simulink model "Schloss_Alarm_Box"  (R2019b)
settings: Solver=FixedStepAuto  StartTime=0.0  StopTime=10.0  RelTol=1e-3
PreLoadFcn:
  | waijung.modelPreload; % Required for working with Waijung Blockset. Do not remove.
undefined symbols (not defined in the file): HSEOSC, Link, LQFP176, ST, STM32F417IG
libraries: canmsglib x8, stm32f4_canbus_lib x4, simulink x2, stm32f4_io_lib x2, stm32f4_device_config_lib x1
CloseFcn:
  | waijung.modelClose; % Required for working with Waijung Blockset. Do not remove.
settings Model: Creator=id605605  LastModifiedBy=MichaelRogalski
settings OptimizationCC: DefaultParameterBehavior=Inlined  EnhancedBackFolding=on  PassReuseOutputArgsAs=Individual arguments  ZeroExternalMemoryAtStartup=off  ZeroInternalMemoryAtStartup=off  OptimizeBlockOrder=speed  DifferentSizesBufferReuse=on  OptimizationCustomize=off  EfficientTunableParamExpr=on
settings DebuggingCC: ParameterTunabilityLossMsg=error  ArithmeticOperatorsInVariantConditions=warning
settings HardwareCC: ProdBitPerPointer=32  ProdBitPerSizeT=32  ProdBitPerPtrDiffT=32  ProdLargestAtomicFloat=None  ProdIntDivRoundTo=Undefined  ProdWordSize=32  ProdHWDeviceType=ARM Compatible->Cortex - M4  TargetEndianess=LittleEndian  TargetHWDeviceType=ARM Compatible->Cortex - M4
settings SFSimCC: MATLABDynamicMemAlloc=off  CustomCodeUndefinedFunction=UseInterfaceOnly
settings RTWCC: Description=STM32F4 Target  SystemTargetFile=stm32f4.tlc  GenerateMakefile=off  TemplateMakefile=ert_default_tmf  GenerateReport=on  IncludeHyperlinkInReport=on  LaunchReport=on  GenerateTraceInfo=on  GenerateTraceReport=on  GenerateTraceReportSl=on  GenerateTraceReportSf=on  GenerateTraceReportEml=on
settings CodeAppCC: ForceParamTrailComments=on  IgnoreCustomStorageClasses=off  OperatorAnnotations=on  SimulinkDataObjDesc=on  SFDataObjDesc=on  InsertBlockDesc=on
settings STFCustomTargetCC: TargetLangStandard=C99 (ISO)  MultiwordLength=256  ModelReferenceCompliant=off  CombineOutputUpdateFcns=on  ERTCustomFileBanners=on  SupportContinuousTime=off  SupportNonInlinedSFcns=off  RemoveResetFunc=on  MATLABClassNameForMDSCustomization=Simulink.SoftwareTarget.ERTCustomization  SystemTargetFile=stm32f4.tlc
settings ERTTargetCC: TargetLangStandard=C99 (ISO)  ModelReferenceCompliant=off  ParMdlRefBuildCompliant=off  CompOptLevelCompliant=off  ConcurrentExecutionCompliant=off  ModelStepFunctionPrototypeControlCompliant=off  CPPClassGenCompliant=off  UseToolchainInfoCompliant=off  InlinedParameterPlacement=NonHierarchical  ERTSrcFileBannerTemplate=stm32f4_code_template.cgt  ERTHdrFileBannerTemplate=stm32f4_code_template.cgt  ERTDataSrcFileTemplate=stm32f4_code_template.cgt  ERTDataHdrFileTemplate=stm32f4_code_template.cgt  ERTCustomFileTemplate=stm32f4_file_process.tlc

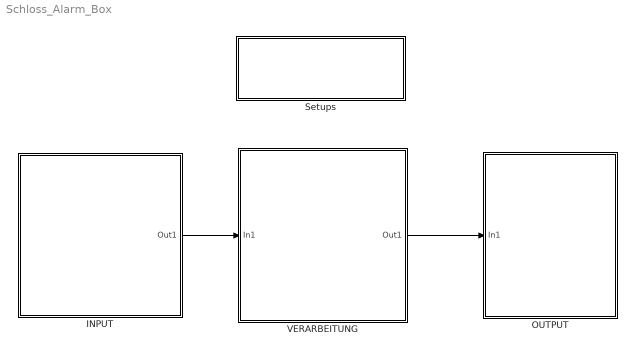
== system Schloss_Alarm_Box ==
  INPUT : Subsystem
  OUTPUT : Subsystem
  Setups : Subsystem
  VERARBEITUNG : Subsystem
  wires:
  INPUT/1(Out1) -> VERARBEITUNG/1(In1)
  VERARBEITUNG/1(Out1) -> OUTPUT/1(In1)

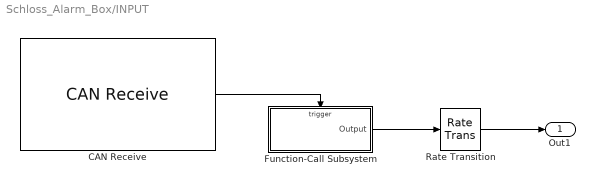
== system Schloss_Alarm_Box/INPUT ==
  CAN Receive : stm32f4_canbus_lib/CAN Receive  conf=Rx  canmodule=1  idtype=Standard  filtertype=Mask  id=0  idmask=0  enableisr=on  usedlc=off  datatype=single  data0type=uint32  data1type=uint32  data2type=Not used  data3type=Not used  data4type=Not used  data5type=Not used  data6type=Not used  data7type=Not used  buffersize=8  sampletime=-1  sampletimestr=-1  blockid=INPUTCANReceive  inputarray=[]  inputlabelarray={}  outputarray=[7]  outputlabelarray={'Call ISR' }  compat=0  confstr=[]
      settings: SourceProductName=Waijung Blockset
  Function-Call Subsystem : Subsystem  TreatAsAtomicUnit=on
  Rate Transition : RateTransition
  Out1 : Outport  VectorParamsAs1DForOutWhenUnconnected=off
  wires:
  CAN Receive/1 -> Function-Call Subsystem/Trigger
  Function-Call Subsystem/1(Output) -> Rate Transition/1
  Rate Transition/1 -> Out1/1

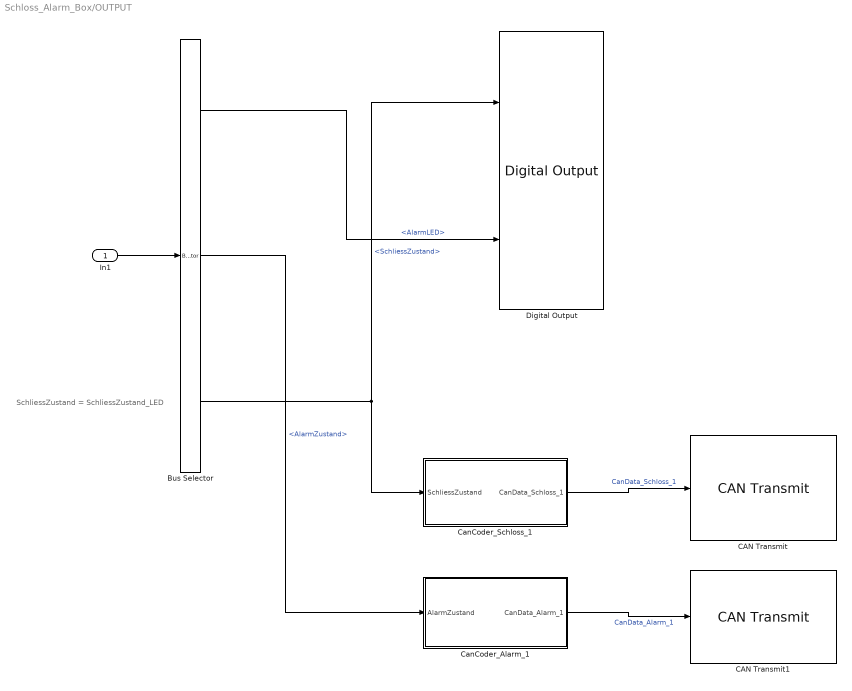
== system Schloss_Alarm_Box/OUTPUT ==
  note: SchliessZustand = SchliessZustand_LED
  In1 : Inport
  Bus Selector : BusSelector  OutputSignals=AlarmLED,AlarmZustand,SchliessZustand
  CAN Transmit : stm32f4_canbus_lib/CAN Transmit  conf=Tx  canmodule=1  transfer=Blocking  timeout=0.005  idtype=Standard  specificid=on  id=25  specificdlc=on  dlc=1  enablestatus=off  datatype=single  data0type=uint8  data1type=Not used  data2type=Not used  data3type=Not used  data4type=Not used  data5type=Not used  data6type=Not used  data7type=Not used  inputarray=[ 3]  inputlabelarray={ 'D0 (uint8)' }  outputarray=[]  outputlabelarray={}  sampletime=-1  sampletimestr=-1  blockid=OUTPUTCANTransmit  compat=0  confstr=[]
  CAN Transmit1 : stm32f4_canbus_lib/CAN Transmit  conf=Tx  canmodule=1  transfer=Blocking  timeout=0.005  idtype=Standard  specificid=on  id=24  specificdlc=on  dlc=1  enablestatus=off  datatype=single  data0type=uint8  data1type=Not used  data2type=Not used  data3type=Not used  data4type=Not used  data5type=Not used  data6type=Not used  data7type=Not used  inputarray=[ 3]  inputlabelarray={ 'D0 (uint8)' }  outputarray=[]  outputlabelarray={}  sampletime=-1  sampletimestr=-1  blockid=OUTPUTCANTransmit1  compat=0  confstr=[]
  CanCoder_Alarm_1 : Subsystem
  CanCoder_Schloss_1 : Subsystem
  Digital Output : stm32f4_io_lib/Digital Output  use_bitband=on  port=C  speed=100  porttype=Push Pull  porttypestr=PP  use_pin0=off  use_pin1=off  use_pin2=on  use_pin3=on  use_pin4=off  use_pin5=off  use_pin6=off  use_pin7=off  use_pin8=off  use_pin9=off  use_pin10=off  use_pin11=off  use_pin12=off  use_pin13=off  use_pin14=off  use_pin15=off  pinstr=GPIO_Pin_2 | GPIO_Pin_3  usedpinarray="[0  0  1  1  0  0  0  0  0  0  0  0  0  0  0  0]"  bitbandingstr=|  sampletime=-1  sampletimestr=-1  blockid=OUTPUTDigitalOutput  enablecustomportlabel=off  globalinit=off  cinputportlabel=In1, In2  coutputportlabel=0
      | #define OUTPUTDigitalOutput_C2 Peripheral_BB(GPIOC->ODR, 2)  /* Output pin */
      | #define OUTPUTDigitalOutput_C3 Peripheral_BB(GPIOC->ODR, 3)  /* Output pin */
      settings: SourceProductName=Waijung Blockset
  wires:
  In1/1 -> Bus Selector/1
  Bus Selector/1 -> Digital Output/2  "<AlarmLED>"
  Bus Selector/2 -> CanCoder_Alarm_1/1(AlarmZustand)  "<AlarmZustand>"
  Bus Selector/3 -> Digital Output/1, CanCoder_Schloss_1/1(SchliessZustand)  "<SchliessZustand>"
  CanCoder_Schloss_1/1(CanData_Schloss_1) -> CAN Transmit/1  "CanData_Schloss_1"
  CanCoder_Alarm_1/1(CanData_Alarm_1) -> CAN Transmit1/1  "CanData_Alarm_1"

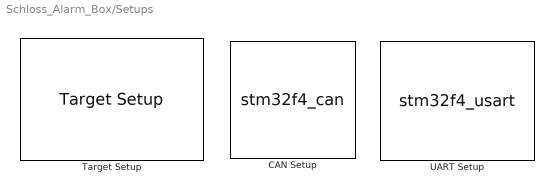
== system Schloss_Alarm_Box/Setups ==
  CAN Setup : S-Function  FunctionName=stm32f4_can  Parameters=conf,canmodule,0,inputarray,outputarray,'','',confstr,sampletime,sampletimestr,blockid  SFunctionDeploymentMode=off  EnableBusSupport=off  mask(stm32f4_can){conf=Setup, canmodule=1, advance=off, bitrate_select=500000, sjw=1tq, bs1=14tq, bs2=6tq, timingconf=Prescaler, brp=4, bitrate=500000, tq=9.5238e-08, autoretransmission=Disable, remaptxpin=A12, remaprxpin=A11, sampletime=-1, sampletimestr=-1, blockid=SetupsCANSetup, inputarray=[], inputlabelarray={}, outputarray=[], outputlabelarray={}, compat=0, confstr=[], presc=4, txportstr=A, txpinstr=12, rxportstr=A, rxpinstr=11, lastmodule=1}
      mask prompts: conf "Configuration"; canmodule "CAN Module"; advance "Advance configuration"; bitrate_select "Baud rate (bps)"; sjw "Resync Jump Width (SJW)"; bs1 "Bit segment 1 (BS1) + PROP_SEG"; bs2 "Bit segment 2 (BS2)"; timingconf "Adjust"; brp "Baud rate prescaler (BRP)"; bitrate "Baud rate (bps)"; tq "Time Quantum (Second), tq"; autoretransmission "Auto Re-transmission"; remaptxpin "CAN Tx pin"; remaprxpin "CAN Rx pin"; sampletime "Sample time (sec)"; sampletimestr "Compiled sample time (sec) in string"; inputarray "Input port"; inputlabelarray "Input port label"; outputarray "Output port"; outputlabelarray "Output port label"; compat "Compatibility (Reserved for future use)"; confstr "Configuration String"; presc "Prescale"; txportstr "Tx port string"; txpinstr "Tx pin string"; rxportstr "Rx port string"; rxpinstr "Rx pin string"; lastmodule "Last module selected"
      mask help:
      | This block setups CAN Module.
      |
      | Auto Re-transmission,
      |  - Enable: The CAN hardware will automatically retransmit the message until it has been
      | successfully transmitted according to the CAN standard.
      |  - Disable: A message will be transmitted only once, independently of the transmission result
      | (successful, error or arbitration lost).
      mask init:
      | stm32f4_can_callback('init');
      mask Help: web(fullfile(waijungdocroot,'stm32f4_can_setup.htm'), '-browser')
      mask TypeOptions conf: Setup
      mask TypeOptions canmodule: 1 | 2
      mask Callback canmodule: stm32f4_can_callback('canmodule');
      mask Callback advance: stm32f4_can_callback('advance');
      mask TypeOptions bitrate_select: 125000 | 250000 | 500000 | 1000000
      mask Callback bitrate_select: stm32f4_can_callback('bitrate_select');
      mask TypeOptions sjw: 1tq | 2tq | 3tq | 4tq
      mask TypeOptions bs1: 1tq | 2tq | 3tq | 4tq | 5tq | 6tq | 7tq | 8tq | 9tq | 10tq | 11tq | 12tq | 13tq | 14tq | 15tq | 16tq
      mask Callback bs1: stm32f4_can_callback('timingconf');
      mask TypeOptions bs2: 1tq | 2tq | 3tq | 4tq | 5tq | 6tq | 7tq | 8tq
      mask Callback bs2: stm32f4_can_callback('timingconf');
      mask TypeOptions timingconf: Prescaler | Baudrate
      mask Callback timingconf: stm32f4_can_callback('timingconf');
      mask Callback brp: stm32f4_can_callback('timingconf');
      mask Callback bitrate: stm32f4_can_callback('timingconf');
      mask TypeOptions autoretransmission: Enable | Disable
      mask TypeOptions remaptxpin: Not used | A12 | B9 | D1 | H13
      mask Callback remaptxpin: stm32f4_can_callback('remaptxpin');
      mask TypeOptions remaprxpin: Not used | A11 | B8 | D0 | I9
      mask Callback remaprxpin: stm32f4_can_callback('remaprxpin');
      mask Callback sampletime: stm32f4_can_callback('sampletime');
      mask Callback sampletimestr: stm32f4_can_callback('sampletimestr');
      mask Callback blockid: stm32f4_can_callback('blockid');
      mask Display: text(0.5, 0.5, 'CAN1_Setup\nSpeed (bps): 500000\nTx/Rx pin: A12/A11','ver','middle','hor','center');
  Target Setup : stm32f4_device_config_lib/Target Setup  Priority=100  compiler=GNU ARM  previous_compiler=GNU ARM  mcu=STM32F417IG (LQFP176)  mcustr=STM32F417IG  clockconfig=HSEOSC-8MHz  system_stm32f4xx_c_path=D:\Downloads\waijung17_03a\targets\stm32f4_target\stm32f4\utils\system_stm32f4xx_default\STM32F40_41xxx\hseosc8mhz  showmemoryconfiguration=off  stacksize=0x2000  heapsize=0x2000  enableautocompiledownload=on  fullchiperase=off  programmerinterface=ST-Link  editctrlstr=on  compilercontrolstr=$(patsubst %, -I%, .) -mcpu=cortex-m4 -mthumb -mthumb-interwork -mfloat-abi=hard -mfpu=fpv4-sp-d16 -ffast-math -Wall -Wextra -Ofast  assemblercontrolstr=$(patsubst %, -I%, .) -mcpu=cortex-m4 -mthumb -mthumb-interwork -mfloat-abi=hard -mfpu=fpv4-sp-d16 -ffast-math -Wall -Wextra -Ofast -Wa,-amhls=$(<:.s=.lst) -D__STACK_SIZE=$(STACK_SIZE) -D__HEAP_SIZE=$(HEAP_SIZE)  linkercontrolstr=-T$(LD_SCRIPT) -g -Wl,-Map=$(MAP),--cref,--no-warn-mismatch -mcpu=cortex-m4 -mthumb -mthumb-interwork -mfloat-abi=hard -mfpu=fpv4-sp-d16 -specs=nosys.specs  runafterdownload=on  execprofile=None  profileruart=3  profilerbaud=500000  profilertxpin=D8  profilerinitstr=0.01,168000000,1680000,500000,0  manualsetsampletime=off  sampletime=0.01  blockid=SetupsTargetSetup  systickreloadvalue=1680000  hseval=8000000  lastprofileruart=3  hclk=168000000  flashorigin=0x8000000  flashlength=1024k  ramorigin=0x20000000  ramlength=128k  useextram=off
      settings: SourceProductName=Waijung Blockset
  UART Setup : S-Function  Priority=1  FunctionName=stm32f4_usart  Parameters=configuration,uartmodule,transfer,baudrate,inputtype,outputtype,confstr,binheaderarray,binterminatorarray,asciiheader,asciiterminator,bindatalength,packetmode,varname,sampletime,sampletimestr,blockid  SFunctionDeploymentMode=off  EnableBusSupport=off  mask(stm32f4_usart){configuration=Setup, uartmodule=2, baudrate=115200, databits=8, parity=No, stopbit=1, remaptxpin=A2, remaprxpin=A3, flowcontrol=None, remapctspin=Not used, remaprtspin=Not used, advanceoptions=off, rxbuffersize=512, txbuffersize=512, transfer=Blocking, packetmode=Ascii, binheader='7E 7E', binterminator='03 03', porttype_double=1, porttype_single=0, porttype_int8=1, porttype_uint8=0, porttype_int16=0, porttype_uint16=0, porttype_int32=0, porttype_uint32=0, asciiformat='%d,%f', rx_asciiterminator=CRLF (0x0D 0x0A - "\r\n"), tx_asciiterminator=CR (0x0D - "\r"), storagename=<empty>, varname=, inputtype=[0], outputtype=[0], binheaderarray=[0], binterminatorarray=[0], bindatalength=0, asciiheader='', asciiterminator=[0], sampletime=-1, sampletimestr=-1, blockid=SetupsUARTSetup, confstr=[ "dummy", "1", "A", "2", "1", "A", "3", "0", "*", "*", "0", "*", "*", "1", "4", "6", "1", "4", "5", "512", "512", "1", "2", "115200", "8", "No", "1", "None", "USART2"], lastmodule=2}
      mask prompts: uartmodule "UART Module"; baudrate "Baud rate (bps)"; databits "Data bits"; stopbit "Stop bit"; remaptxpin "Tx Pin"; remaprxpin "Rx Pin"; flowcontrol "Hardware flow control"; remapctspin "HW Flow control, CTS Pin"; remaprtspin "HW Flow control, RTS Pin"; advanceoptions "Advance options"; rxbuffersize "Rx buffer size (bytes)"; txbuffersize "Tx buffer size (bytes)"; packetmode "Packet mode"; binheader "Binary header (example: '7E 7E')"; binterminator "Binary terminator (example: '03 03')"; porttype_double "Number of data port, type DOUBLE"; porttype_single "Number of data port, type SINGLE"; porttype_int8 "Number of data port, type INT8"; porttype_uint8 "Number of data port, type UINT8"; porttype_int16 "Number of data port, type INT16"; porttype_uint16 "Number of data port, type UINT16"; porttype_int32 "Number of data port, type INT32"; porttype_uint32 "Number of data port, type UINT32"; asciiformat "Ascii format"; rx_asciiterminator "End of packet"; tx_asciiterminator "End of packet"; storagename "Buffer"; varname "Var name"; inputtype "Input data type"; outputtype "Output data type"; binheaderarray "Binary header"; binterminatorarray "Binary terminator"; bindatalength "Binary data length"; asciiheader "Ascii header (printf format)"; asciiterminator "Ascii terminator"; sampletime "Sample time (sec)"; sampletimestr "Compiled sample time (sec) in string"; confstr "Configuration string"; lastmodule "Last module selected"
      mask help:
      | Default STM32F4DISCOVERY + aMG F4 Connect 2 + aMG USB Converter N2 settings use
      |
      | USART3, Tx D8, Rx D9 and USB Serial Converter A.
      mask init:
      | stm32f4_usart_callback('init');
      mask Help: web(fullfile(waijungdocroot,'stm32f4_usart_setup.htm'), '-browser')
      mask TypeOptions configuration: Setup | Tx | Rx
      mask Callback configuration: stm32f4_usart_callback('configuration');
      mask TypeOptions uartmodule: 1 | 2 | 3 | 4 | 5 | 6
      mask Callback uartmodule: stm32f4_usart_callback('uartmodule');
      mask Callback baudrate: stm32f4_usart_callback('baudrate');
      mask TypeOptions databits: 8
      mask TypeOptions parity: No | Odd | Even
      mask TypeOptions stopbit: 0.5 | 1 | 1.5 | 2
      mask TypeOptions remaptxpin: Not used | A2 | D5
      mask TypeOptions remaprxpin: Not used | A3 | D6
      mask TypeOptions flowcontrol: None | RTS | CTS | RTS/CTS
      mask Callback flowcontrol: stm32f4_usart_callback('flowcontrol');
      mask TypeOptions remapctspin: Not used | A0 | D3
      mask TypeOptions remaprtspin: Not used | A1 | D4
      mask Callback advanceoptions: stm32f4_usart_callback('advanceoptions');
      mask TypeOptions rxbuffersize: 16 | 32 | 64 | 128 | 256 | 512 | 1024 | 2048
      mask TypeOptions txbuffersize: 16 | 32 | 64 | 128 | 256 | 512 | 1024 | 2048
      mask TypeOptions transfer: Blocking | Non-Blocking
      mask Callback transfer: stm32f4_usart_callback('transfer');
      mask TypeOptions packetmode: Ascii | Binary | String Buffer
      mask Callback packetmode: stm32f4_usart_callback('packetmode');
      mask Callback binheader: stm32f4_usart_callback('binheader');
      mask Callback binterminator: stm32f4_usart_callback('binterminator');
      mask Callback porttype_double: stm32f4_usart_callback('porttype');
      mask Callback porttype_single: stm32f4_usart_callback('porttype');
      mask Callback porttype_int8: stm32f4_usart_callback('porttype');
      mask Callback porttype_uint8: stm32f4_usart_callback('porttype');
      mask Callback porttype_int16: stm32f4_usart_callback('porttype');
      mask Callback porttype_uint16: stm32f4_usart_callback('porttype');
      mask Callback porttype_int32: stm32f4_usart_callback('porttype');
      mask Callback porttype_uint32: stm32f4_usart_callback('porttype');
      mask Callback asciiformat: stm32f4_usart_callback('asciiformat');
      mask TypeOptions rx_asciiterminator: CR (0x0D - "\r") | LF (0x0A - "\n") | CRLF (0x0D 0x0A - "\r\n")
      mask Callback rx_asciiterminator: stm32f4_usart_callback('rx_asciiterminator');
      mask TypeOptions tx_asciiterminator: CR (0x0D - "\r") | LF (0x0A - "\n") | CRLF (0x0D 0x0A - "\r\n") | None
      mask Callback tx_asciiterminator: stm32f4_usart_callback('tx_asciiterminator');
      mask TypeOptions storagename: <empty>
      mask Callback storagename: stm32f4_usart_callback('storagename');
      mask Callback varname: stm32f4_usart_callback('varname');
      mask Callback sampletime: stm32f4_usart_callback('sampletime');
      mask Callback sampletimestr: stm32f4_usart_callback('sampletimestr');
      mask Callback blockid: stm32f4_usart_callback('blockid');
      mask Display: text(0.5, 0.5, 'Module: USART2_Setup\nBaud (Bps): 115200\nDMA Buffer: 512/512\nTx/Rx Pin: A2/A3','ver','middle','hor','center');

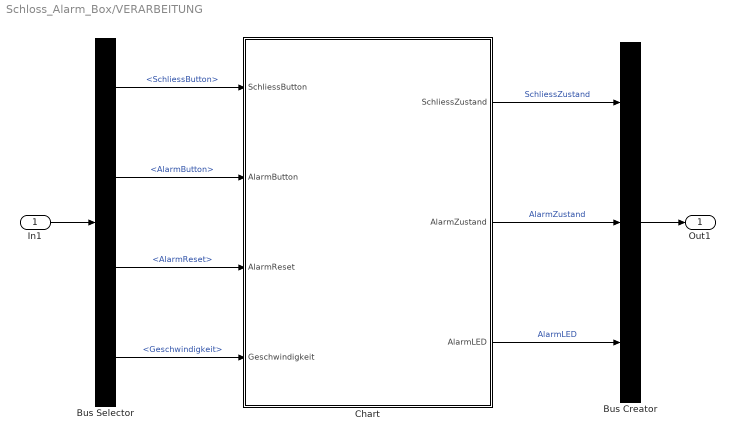
== system Schloss_Alarm_Box/VERARBEITUNG ==
  In1 : Inport
  Bus Creator : BusCreator  Inputs=3
  Bus Selector : BusSelector  OutputSignals=SchliessButton,AlarmButton,AlarmReset,Geschwindigkeit
  Chart : Stateflow chart  TreatAsAtomicUnit=on
  Out1 : Outport  VectorParamsAs1DForOutWhenUnconnected=off
  wires:
  Bus Creator/1 -> Out1/1
  In1/1 -> Bus Selector/1
  Chart/1(SchliessZustand) -> Bus Creator/1  "SchliessZustand"
  Chart/2(AlarmZustand) -> Bus Creator/2  "AlarmZustand"
  Chart/3(AlarmLED) -> Bus Creator/3  "AlarmLED"
  Bus Selector/1 -> Chart/1(SchliessButton)  "<SchliessButton>"
  Bus Selector/2 -> Chart/2(AlarmButton)  "<AlarmButton>"
  Bus Selector/3 -> Chart/3(AlarmReset)  "<AlarmReset>"
  Bus Selector/4 -> Chart/4(Geschwindigkeit)  "<Geschwindigkeit>"

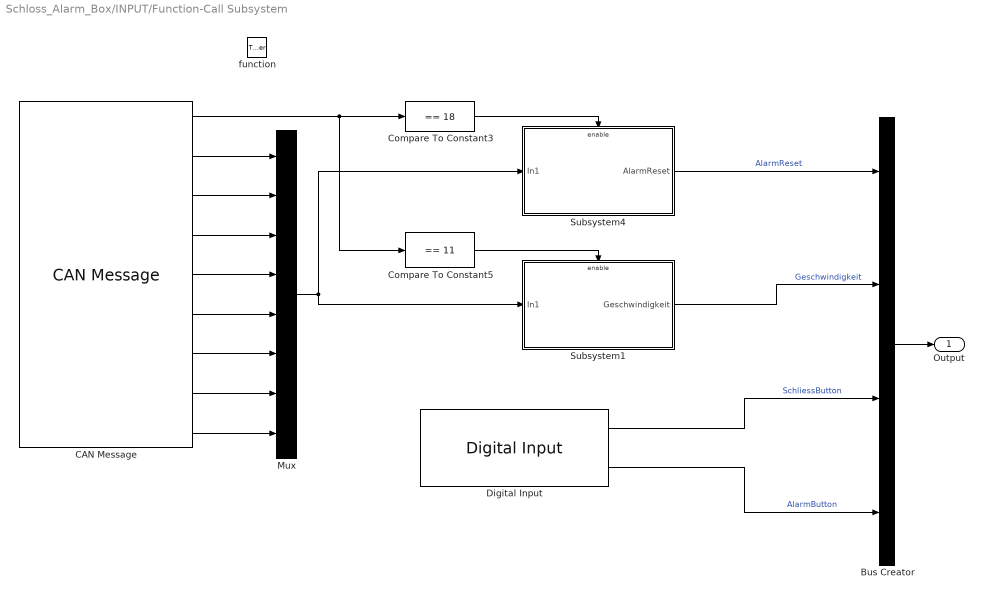
== system Schloss_Alarm_Box/INPUT/Function-Call Subsystem ==
  function : TriggerPort  TriggerType=function-call  VariantControl=Variant
  Bus Creator : BusCreator  Inputs=4
  CAN Message : stm32f4_canbus_lib/CAN Message  conf=Msg  canmodule=1  usedlc=off  datatype=double  data0type=uint8  data1type=uint8  data2type=uint8  data3type=uint8  data4type=uint8  data5type=uint8  data6type=uint8  data7type=uint8  sampletime=-1  sampletimestr=-1  blockid=INPUTFunctionCallSubsystemCANMessage  inputarray=[]  inputlabelarray={}  outputarray=[ 7, 3, 3, 3, 3, 3, 3, 3, 3]  outputlabelarray={'ID', 'D0 (uint8)', 'D1 (uint8)', 'D2 (uint8)', 'D3 (uint8)', 'D4 (uint8)', 'D5 (uint8)', 'D6 (uint8)', 'D7 (uint8)' }  compat=0  confstr=[]
      settings: SourceProductName=Waijung Blockset
  Compare To Constant3 : simulink/Logic and Bit Operations/Compare To Constant  relop===  const=18  OutDataTypeStr=boolean
  Compare To Constant5 : simulink/Logic and Bit Operations/Compare To Constant  relop===  const=11  OutDataTypeStr=boolean
  Digital Input : stm32f4_io_lib/Digital Input  port=C  speed=100  porttype=None  porttypestr=NOPULL  use_pin0=on  use_pin1=on  use_pin2=off  use_pin3=off  use_pin4=off  use_pin5=off  use_pin6=off  use_pin7=off  use_pin8=off  use_pin9=off  use_pin10=off  use_pin11=off  use_pin12=off  use_pin13=off  use_pin14=off  use_pin15=off  pinstr=GPIO_Pin_0 | GPIO_Pin_1  usedpinarray="[1  1  0  0  0  0  0  0  0  0  0  0  0  0  0  0]"  bitbandingstr=|  sampletime=-1  sampletimestr=-1  blockid=INPUTFunctionCallSubsystemDigitalInput  enablecustomportlabel=off  glabalinit=off  cinputportlabel=In1, In2  coutputportlabel=Out1, Out2
      | #define INPUTFunctionCallSubsystemDigitalInput_A0 Peripheral_BB(GPIOA->IDR, 0)  /* Output pin */
      | #define INPUTFunctionCallSubsystemDigitalInput_A1 Peripheral_BB(GPIOA->IDR, 1)  /* Output pin */
  Mux : Mux  Inputs=8
  Subsystem1 : Subsystem
  Subsystem4 : Subsystem
  Output : Outport  VectorParamsAs1DForOutWhenUnconnected=off
  wires:
  CAN Message/1 -> Compare To Constant5/1, Compare To Constant3/1
  CAN Message/3 -> Mux/2
  CAN Message/2 -> Mux/1
  CAN Message/4 -> Mux/3
  CAN Message/5 -> Mux/4
  CAN Message/6 -> Mux/5
  CAN Message/7 -> Mux/6
  CAN Message/8 -> Mux/7
  CAN Message/9 -> Mux/8
  Bus Creator/1 -> Output/1
  Compare To Constant3/1 -> Subsystem4/Enable
  Mux/1 -> Subsystem4/1(In1), Subsystem1/1(In1)
  Compare To Constant5/1 -> Subsystem1/Enable
  Subsystem4/1(AlarmReset) -> Bus Creator/1  "AlarmReset"
  Subsystem1/1(Geschwindigkeit) -> Bus Creator/2  "Geschwindigkeit"
  Digital Input/1 -> Bus Creator/3  "SchliessButton"
  Digital Input/2 -> Bus Creator/4  "AlarmButton"

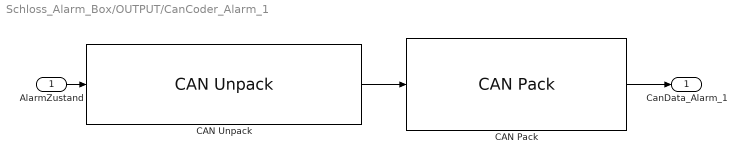
== system Schloss_Alarm_Box/OUTPUT/CanCoder_Alarm_1 ==
  AlarmZustand : Inport
  CAN Pack : canmsglib/CAN Pack  MsgList=(none)  MsgName=CAN Msg  MsgIDType=Standard (11-bit identifier)  MsgIdentifier=24  MsgLength=1  Remote=off  ApplyMinMax=off  BusOutput=off  SignalInfo="{  }"
      settings: SourceProductName=Simulink Real-Time  SourceProductBaseCode=XP  DataFormat=raw data
  CAN Unpack : canmsglib/CAN Unpack  MsgList=(none)  MsgName=CAN_Data_Alarm1  MsgIDType=Standard (11-bit identifier)  MsgIdentifier=24  MsgLength=1  SignalInfo={ 'AlarmZustand', '0', '1', 'LE', 'unsigned', 'Standard', '0', '1', '0', '-Inf', 'Inf' }  IDPort=off  TimestampPort=off  ErrorPort=off  RemotePort=off  LengthPort=off  StatusPort=off  ApplyMinMax=off
      settings: SourceProductName=Simulink Real-Time  SourceProductBaseCode=XP
  CanData_Alarm_1 : Outport  VectorParamsAs1DForOutWhenUnconnected=off
  wires:
  CAN Unpack/1 -> CAN Pack/1
  CAN Pack/1 -> CanData_Alarm_1/1
  AlarmZustand/1 -> CAN Unpack/1

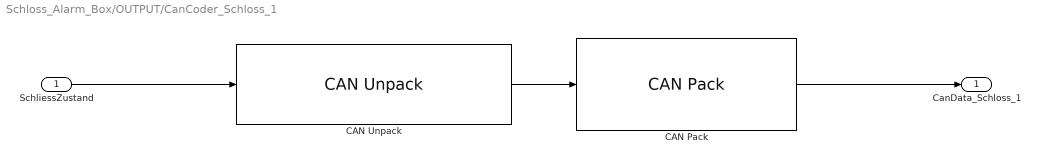
== system Schloss_Alarm_Box/OUTPUT/CanCoder_Schloss_1 ==
  SchliessZustand : Inport
  CAN Pack : canmsglib/CAN Pack  MsgList=(none)  MsgName=CAN Msg  MsgIDType=Standard (11-bit identifier)  MsgIdentifier=25  MsgLength=1  Remote=off  ApplyMinMax=off  BusOutput=off  SignalInfo={}
      settings: SourceProductName=Simulink Real-Time  SourceProductBaseCode=XP  DataFormat=raw data
  CAN Unpack : canmsglib/CAN Unpack  MsgList=(none)  MsgName=CAN_Data_Schloss1  MsgIDType=Standard (11-bit identifier)  MsgIdentifier=25  MsgLength=1  SignalInfo={ 'SchlossZustand', '0', '1', 'LE', 'unsigned', 'Standard', '0', '1', '0', '-Inf', 'Inf' }  IDPort=off  TimestampPort=off  ErrorPort=off  RemotePort=off  LengthPort=off  StatusPort=off  ApplyMinMax=off
      settings: SourceProductName=Simulink Real-Time  SourceProductBaseCode=XP
  CanData_Schloss_1 : Outport  VectorParamsAs1DForOutWhenUnconnected=off
  wires:
  CAN Pack/1 -> CanData_Schloss_1/1
  CAN Unpack/1 -> CAN Pack/1
  SchliessZustand/1 -> CAN Unpack/1

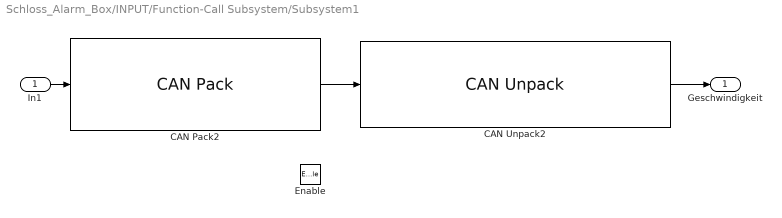
== system Schloss_Alarm_Box/INPUT/Function-Call Subsystem/Subsystem1 ==
  In1 : Inport
  Enable : EnablePort
  CAN Pack2 : canmsglib/CAN Pack  MsgList=(none)  MsgName=CAN_Data_Bremse2  MsgIDType=Standard (11-bit identifier)  MsgIdentifier=11  MsgLength=1  Remote=off  ApplyMinMax=off  BusOutput=off  SignalInfo={}
      settings: SourceProductName=Simulink Real-Time  SourceProductBaseCode=XP  DataFormat=raw data
  CAN Unpack2 : canmsglib/CAN Unpack  MsgList=(none)  MsgName=CAN_Data_Bremse2  MsgIDType=Standard (11-bit identifier)  MsgIdentifier=11  MsgLength=1  SignalInfo={'Geschwindigkeit','0','8','LE','unsigned','Standard','0','1','0','-Inf','Inf'}  IDPort=off  TimestampPort=off  ErrorPort=off  RemotePort=off  LengthPort=off  StatusPort=off  ApplyMinMax=off
      settings: SourceProductName=Simulink Real-Time  SourceProductBaseCode=XP
  Geschwindigkeit : Outport  VectorParamsAs1DForOutWhenUnconnected=off
  wires:
  CAN Pack2/1 -> CAN Unpack2/1
  In1/1 -> CAN Pack2/1
  CAN Unpack2/1 -> Geschwindigkeit/1

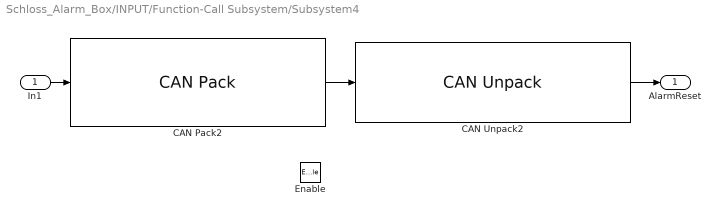
== system Schloss_Alarm_Box/INPUT/Function-Call Subsystem/Subsystem4 ==
  In1 : Inport
  Enable : EnablePort
  CAN Pack2 : canmsglib/CAN Pack  MsgList=(none)  MsgName=CAN_Data_Cockpit3  MsgIDType=Standard (11-bit identifier)  MsgIdentifier=18  MsgLength=1  Remote=off  ApplyMinMax=off  BusOutput=off  SignalInfo={}
      settings: SourceProductName=Simulink Real-Time  SourceProductBaseCode=XP  DataFormat=raw data
  CAN Unpack2 : canmsglib/CAN Unpack  MsgList=(none)  MsgName=CAN_Data_Schloss1  MsgIDType=Standard (11-bit identifier)  MsgIdentifier=18  MsgLength=1  SignalInfo={'AlarmReset','0','1','LE','unsigned','Standard','0','1','0','-Inf','Inf'}  IDPort=off  TimestampPort=off  ErrorPort=off  RemotePort=off  LengthPort=off  StatusPort=off  ApplyMinMax=off
      settings: SourceProductName=Simulink Real-Time  SourceProductBaseCode=XP
  AlarmReset : Outport  VectorParamsAs1DForOutWhenUnconnected=off
  wires:
  CAN Unpack2/1 -> AlarmReset/1
  In1/1 -> CAN Pack2/1
  CAN Pack2/1 -> CAN Unpack2/1

== stateflow chart Schloss_Alarm_Box/VERARBEITUNG/Chart ==
  state State_Geschlossen
    en, du: SchliessZustand = true
    state State_AA_OFF
    state State_AA_ON
      state State_TRIGGER_ON
        en, du: AlarmZustand = true
        AlarmLED = true
      state State_TRIGGER_OFF
        state State_AlarmLED_OFF
          en, du: AlarmLED = false
        state State_AlarmLED_ON
          en, du: AlarmLED = true
        State_AlarmLED_OFF -> State_AlarmLED_ON : [after(0.5, sec)]
        (default) -> State_AlarmLED_ON
        State_AlarmLED_ON -> State_AlarmLED_OFF : [AlarmZustand == false && after(0.5, sec)]
      State_TRIGGER_OFF -> State_TRIGGER_ON : [AlarmButton == true]
      (default) -> State_TRIGGER_OFF
    (default) -> State_AA_OFF
    State_AA_OFF -> State_AA_ON : [Geschwindigkeit == 0]
    State_AA_ON -> State_AA_OFF : [Geschwindigkeit > 0]
  state State_Offen
    en, du: SchliessZustand = false
    state State_AlarmReset_Gedrueckt
      en, du: AlarmZustand = false
      AlarmLED = false
    state State_AlarmReset_NichtGedrueckt
    State_AlarmReset_NichtGedrueckt -> State_AlarmReset_Gedrueckt : [AlarmReset == true]
    (default) -> State_AlarmReset_NichtGedrueckt
  (default) -> State_Offen : {AlarmZustand = false}
  State_Offen -> State_Geschlossen : [SchliessButton == true && after(0.5,sec)]
  State_Geschlossen -> State_Offen [order 2] : [SchliessButton == true && after(0.5,sec)]
  State_Geschlossen -> State_Offen [order 1] : [SchliessButton == true && AlarmZustand == false && after(0.5,sec)]{AlarmLED = false}
  data: SchliessButton input; AlarmButton input; SchliessZustand output boolean; AlarmZustand output boolean; AlarmReset input; Geschwindigkeit input; AlarmLED output boolean
  events: AlarmResetUpdated local FUNCTION_CALL_EVENT
